simulink model "Problem_1"  (R2020a)
settings: Solver=VariableStepAuto  StartTime=0.0  StopTime=70  RelTol=1e-3
settings Model: PauseTimes=10  Creator=Admin  LastModifiedBy=Admin

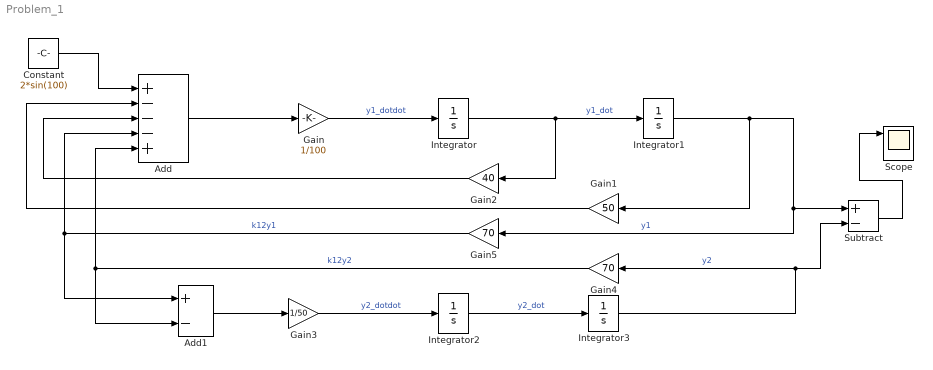
== system Problem_1 ==
  Add : Sum  Inputs=+---+
  Add1 : Sum  Inputs=+-
  Constant : Constant  Value=2*sin(100)
  Gain : Gain  Gain=1/100
  Gain1 : Gain  Gain=50
  Gain2 : Gain  Gain=40
  Gain3 : Gain  Gain=1/50
  Gain4 : Gain  Gain=70
  Gain5 : Gain  Gain=70
  Integrator{,1..3} (4 alike) : Integrator
  Scope : Scope  NumInputPorts=3
  Subtract : Sum  Inputs=+-
  wires:
  Integrator/1 -> Gain2/1, Integrator1/1  "y1_dot"
  Gain/1 -> Integrator/1  "y1_dotdot"
  Integrator1/1 -> Gain1/1, Subtract/1, Gain5/1  "y1"
  Integrator2/1 -> Integrator3/1  "y2_dot"
  Gain3/1 -> Integrator2/1  "y2_dotdot"
  Integrator3/1 -> Subtract/2, Gain4/1  "y2"
  Add/1 -> Gain/1
  Constant/1 -> Add/1
  Gain1/1 -> Add/2
  Gain2/1 -> Add/3
  Gain5/1 -> Add1/1, Add/4  "k12y1"
  Gain4/1 -> Add1/2, Add/5  "k12y2"
  Add1/1 -> Gain3/1
  Subtract/1 -> Scope/1
